simulink library "tether000_cl"  (R2018b)
settings: Solver=VariableStepAuto  StartTime=0.0  StopTime=10.0  RelTol=1e-3
undefined symbols (not defined in the file or in its folder): thr
libraries: NNodeTether_cl x1, twoNodeTether_cl x1
settings Model: Creator=mcobb  LastModifiedBy=mcobb

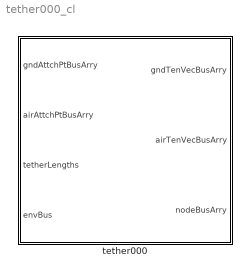
== system tether000_cl ==
  tether000 : Subsystem  mask{thr=thr}
      mask prompts: thr "Tether parameter structure"
      mask help:
      | Tether parameters structure where each element must have the fields
      | thr.N                        = Number of nodes per tether (all elements must have the same value)
      | thr(i).diameter        = Tether diameter, in meters
      | thr(i).youngsMod   = Youngs modulus
      | thr(i).density           = Density
      | thr(i).dragCoeff        = Drag coefficient
      | thr(i).dampingRatio     = Damping ratio
      | thr(i).fluidDensity     = Fluid Density
      | thr(i).gravAccel        = Acceleration of gravity
      | thr(i).vehicleMass      = Mass of vehicle
      | thr(i).initVhclAttchPt  = Tether attachment point in lifting body coordinate system
      | thr(i).initGndStnAttchPt  = Tether attachment point in ground station coordinate system
      mask init:
      | tether_init
      mask Display:
      | % xPos = linspace(100,400,numel(thr));
      | % centerLine = 250;
      | % offsets = [0 100 -100];
      | % for ii = 1:numel(thr)
      | %     image('tether.png',[centerLine+offsets(ii) 0 323 682]/4)
      | % end
      | 
      | port_label('input',1,'gndAttchPtBusArry')
      | port_label('input',2,'airAttchPtBusArry')
      | port_label('input',3,'tetherLengths')
      | port_label('input',4,'flow')
      | 
      | port_label('output',1,'gndTenVecBusArry')
      | port_label('output',2,'airTenVecBusArry')
      | port_label('output',3,'nodeBusArry')

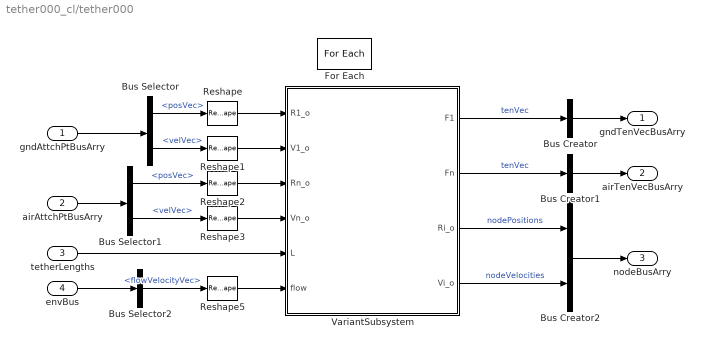
== system tether000_cl/tether000 ==
  gndAttchPtBusArry : Inport  OutDataTypeStr=Bus: thrAttachPtKinematicsBus  Partition=on  PartitionDimension=1  PartitionWidth=1  PartitionOffset=0
  airAttchPtBusArry : Inport  Port=2  OutDataTypeStr=Bus: thrAttachPtKinematicsBus  Partition=on  PartitionDimension=1  PartitionWidth=1  PartitionOffset=0
  tetherLengths : Inport  Port=3  Partition=on  PartitionDimension=1  PartitionWidth=1  PartitionOffset=0
  envBus : Inport  Port=4  OutDataTypeStr=Bus: envBus
  Bus Creator : BusCreator  Inputs=1  OutDataTypeStr=Bus: thrTenVecBus  NonVirtualBus=on
  Bus Creator1 : BusCreator  Inputs=1  OutDataTypeStr=Bus: thrTenVecBus  NonVirtualBus=on
  Bus Creator2 : BusCreator  Inputs=2  OutDataTypeStr=Bus: thrNodeBus  NonVirtualBus=on
  Bus Selector : BusSelector  OutputSignals=posVec,velVec
  Bus Selector1 : BusSelector  OutputSignals=posVec,velVec
  Bus Selector2 : BusSelector  OutputSignals=flowVelocityVec
  For Each : ForEach  DisableCoverage=on  IterateSubsysMaskParameter=on  SubsysMaskParameterIterationDimension=2  IndexMode=One-based
  Reshape{,1..3,5} (5 alike) : Reshape  OutputDimensionality=Column vector (2-D)
  VariantSubsystem : Subsystem  VariantControlMode=Label  Variant=on  LabelModeActiveChoice=VSS_NNodeTether
  gndTenVecBusArry : Outport  ConcatenationDimension=1
  airTenVecBusArry : Outport  Port=2  ConcatenationDimension=1
  nodeBusArry : Outport  Port=3  ConcatenationDimension=1
  wires:
  Bus Creator/1 -> gndTenVecBusArry/1
  Bus Creator1/1 -> airTenVecBusArry/1
  Bus Creator2/1 -> nodeBusArry/1
  envBus/1 -> Bus Selector2/1
  VariantSubsystem/1(F1) -> Bus Creator/1  "tenVec"
  VariantSubsystem/2(Fn) -> Bus Creator1/1  "tenVec"
  VariantSubsystem/3(Ri_o) -> Bus Creator2/1  "nodePositions"
  VariantSubsystem/4(Vi_o) -> Bus Creator2/2  "nodeVelocities"
  airAttchPtBusArry/1 -> Bus Selector1/1
  Bus Selector1/2 -> Reshape3/1  "<velVec>"
  Bus Selector/2 -> Reshape1/1  "<velVec>"
  Bus Selector/1 -> Reshape/1  "<posVec>"
  Bus Selector1/1 -> Reshape2/1  "<posVec>"
  gndAttchPtBusArry/1 -> Bus Selector/1
  Reshape/1 -> VariantSubsystem/1(R1_o)
  Reshape1/1 -> VariantSubsystem/2(V1_o)
  Reshape2/1 -> VariantSubsystem/3(Rn_o)
  Reshape3/1 -> VariantSubsystem/4(Vn_o)
  tetherLengths/1 -> VariantSubsystem/5(L)
  Reshape5/1 -> VariantSubsystem/6(flow)
  Bus Selector2/1 -> Reshape5/1  "<flowVelocityVec>"

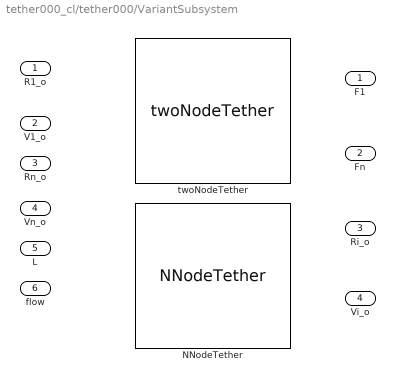
== system tether000_cl/tether000/VariantSubsystem ==
  R1_o : Inport
  V1_o : Inport  Port=2
  Rn_o : Inport  Port=3
  Vn_o : Inport  Port=4
  L : Inport  Port=5
  flow : Inport  Port=6
  NNodeTether : NNodeTether_cl/NNodeTether  SystemSampleTime=-1  VariantControl=VSS_NNodeTether
  twoNodeTether : twoNodeTether_cl/twoNodeTether  SystemSampleTime=-1  VariantControl=VSS_twoNodeTether
  F1 : Outport
  Fn : Outport  Port=2
  Ri_o : Outport  Port=3
  Vi_o : Outport  Port=4
